simulink model "ProximitySensor"  (Simulink 8.7)
settings: Solver=VariableStepAuto  StartTime=0.0  StopTime=10.0  RelTol=1e-3
settings Model: Creator=maximilian  LastModifiedBy=maximilian
settings DataIOCC: LimitDataPoints=off  SaveFormat=Dataset
settings DebuggingCC: UnderspecifiedInitializationDetection=Simplified  MergeDetectMultiDrivingBlocksExec=error
settings HardwareCC: ProdBitPerPointer=64  ProdLargestAtomicFloat=Float  ProdIntDivRoundTo=Zero  ProdEndianess=LittleEndian  ProdWordSize=64  ProdHWDeviceType=Intel->x86-64 (Windows64)
settings ModelReferenceCC: PropagateSignalLabelsOutOfModel=on
settings ConfigComp: CovModelRefEnable=off

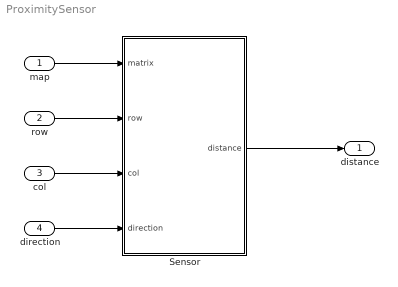
== system ProximitySensor ==
  map : Inport  PortDimensions=[100 100]
  row : Inport  Port=2
  col : Inport  Port=3
  direction : Inport  Port=4
  Sensor : MATLAB Function  TreatAsAtomicUnit=on
  distance : Outport
  wires:
  map/1 -> Sensor/1(matrix)
  col/1 -> Sensor/3(col)
  row/1 -> Sensor/2(row)
  direction/1 -> Sensor/4(direction)
  Sensor/1(distance) -> distance/1

== matlab function Sensor ==
  data: matrix input double; row input double; col input double; distance output double; direction input double
function distance = raycast(matrix, row, col, direction)
    [distance, ~] = TinUtils.raycast(matrix, row, col, direction);
end
